simulink model "task3"  (Simulink 7.5)
settings: Solver=ode3  StartTime=0.0  StopTime=10.0  RelTol=1e-3
settings Model: Creator=Dranik_win  LastModifiedBy=Dranik_win
settings SimEventsCC: propDiagAttribOutput=1  propDiagFcnCallOutput=1  propDiagStatOutput=0

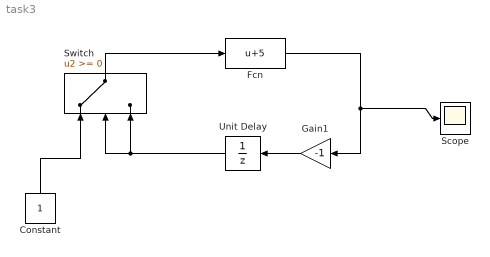
== system task3 ==
  Constant : Constant  OutDataType=fixdt(1, 16)  OutScaling=2^0
  Fcn : Fcn  Expr=u+5  SampleTime=1
  Gain1 : Gain  Gain=-1  ParameterDataType=fixdt(1, 16)  ParameterScaling=2^0  OutDataType=fixdt(1, 16)  OutScaling=2^0
  Scope : Scope
      settings: YMin=-2  YMax=7
  Switch : Switch  OutDataType=fixdt(1, 16)  OutScaling=2^0
  Unit Delay : UnitDelay  SampleTime=-1
  wires:
  Fcn/1 -> Gain1/1, Scope/1
  Gain1/1 -> Unit Delay/1
  Unit Delay/1 -> Switch/2, Switch/3
  Switch/1 -> Fcn/1
  Constant/1 -> Switch/1
